simulink model "controller"  (R2024b)
settings: Solver=FixedStepDiscrete  StartTime=0.0  StopTime=10  FixedStep=1/10  RelTol=1e-3
undefined symbols (not defined in the file or in its folder): MAX_TORQUE, MAX_TORQUE_REVERSE
settings Model: ExtModeTrigDuration=2  Creator=DAUIN-Win10  LastModifiedBy=yoyom
settings SolverCC: AutoInsertRateTranBlk=on
settings OptimizationCC: EnhancedBackFolding=on  PassReuseOutputArgsAs=Individual arguments  ZeroExternalMemoryAtStartup=off  ZeroInternalMemoryAtStartup=off  MaxStackSize=64  OptimizeBlockOrder=speed  DifferentSizesBufferReuse=on  OptimizationCustomize=off  EfficientTunableParamExpr=on
settings DebuggingCC: ParameterTunabilityLossMsg=error  UnconnectedInputMsg=warning  UnconnectedOutputMsg=warning  UnconnectedLineMsg=warning
settings HardwareCC: ProdBitPerInt=16  ProdBitPerPointer=16  ProdBitPerSizeT=16  ProdBitPerPtrDiffT=16  ProdLargestAtomicFloat=None  ProdWordSize=8  ProdHWDeviceType=Atmel->AVR
settings ModelReferenceCC: EnableRefExpFcnMdlSchedulingChecks=on
settings SFSimCC: MATLABDynamicMemAlloc=off
settings RTWCC: Description=Embedded Coder  SystemTargetFile=ert.tlc  HardwareBoard=Arduino Uno  TemplateMakefile=ert_default_tmf  Toolchain=Arduino AVR  BuildConfiguration=Faster Runs  GPUComputeCapability=3.5  DLArmComputeVersion=19.05
settings CodeAppCC: ForceParamTrailComments=on  IgnoreCustomStorageClasses=off  OperatorAnnotations=on  SimulinkDataObjDesc=on  SFDataObjDesc=on  InsertBlockDesc=on
settings ERTTargetCC: SupportContinuousTime=on  SupportNonInlinedSFcns=on  SupportVariableSizeSignals=on  ExtModeTransport=3  ExtModeStaticAlloc=on  ExtModeAutomaticAllocSize=off  ExtModeStaticAllocSize=250  ExtModeMexFile=ext_xcp  ExtModeIntrfLevel=Level2 - Open  InlinedParameterPlacement=Hierarchical  ERTFilePackagingFormat=Compact

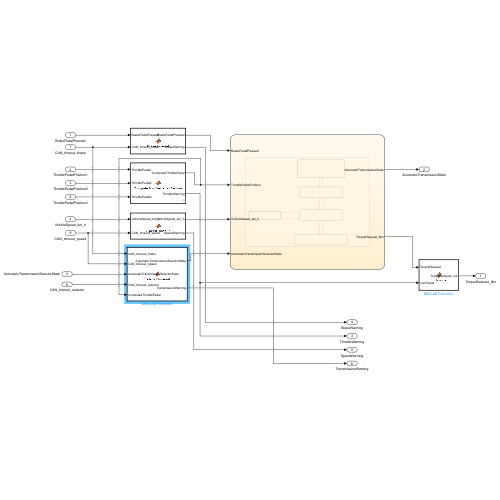
[thumbnail: Simulink's stored preview of the top-level diagram]
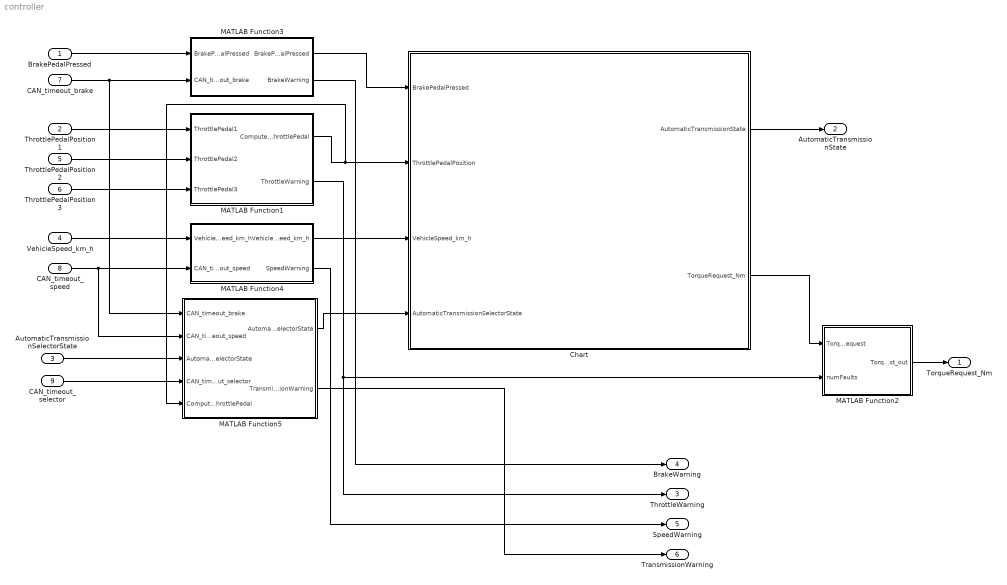
== system controller ==
  BrakePedalPressed : Inport  OutDataTypeStr=boolean
  ThrottlePedalPosition1 : Inport  Port=2  OutDataTypeStr=single
  AutomaticTransmissionSelectorState : Inport  Port=3  OutDataTypeStr=Enum: TransmissionState
  VehicleSpeed_km_h : Inport  Port=4  OutDataTypeStr=single  Unit=km/h
  ThrottlePedalPosition2 : Inport  Port=5  OutDataTypeStr=single
  ThrottlePedalPosition3 : Inport  Port=6  OutDataTypeStr=single
  CAN_timeout_brake : Inport  Port=7
  CAN_timeout_speed : Inport  Port=8
  CAN_timeout_selector : Inport  Port=9
  Chart : Stateflow chart  TreatAsAtomicUnit=on
  MATLAB Function1 : MATLAB Function  TreatAsAtomicUnit=on
  MATLAB Function2 : MATLAB Function  TreatAsAtomicUnit=on
  MATLAB Function3 : MATLAB Function  TreatAsAtomicUnit=on
  MATLAB Function4 : MATLAB Function  TreatAsAtomicUnit=on
  MATLAB Function5 : MATLAB Function  TreatAsAtomicUnit=on
  TorqueRequest_Nm : Outport  OutDataTypeStr=single  Unit=N*m
  AutomaticTransmissionState : Outport  Port=2  OutDataTypeStr=Enum: TransmissionState
  ThrottleWarning : Outport  Port=3  OutDataTypeStr=single  Unit=N*m
  BrakeWarning : Outport  Port=4  OutDataTypeStr=single  Unit=N*m
  SpeedWarning : Outport  Port=5  OutDataTypeStr=single  Unit=N*m
  TransmissionWarning : Outport  Port=6  OutDataTypeStr=single  Unit=N*m
  wires:
  Chart/2(TorqueRequest_Nm) -> MATLAB Function2/1(TorqueRequest)
  Chart/1(AutomaticTransmissionState) -> AutomaticTransmissionState/1
  BrakePedalPressed/1 -> MATLAB Function3/1("BrakePedalPressed ")
  AutomaticTransmissionSelectorState/1 -> MATLAB Function5/3("AutomaticTransmissionSelectorState ")
  VehicleSpeed_km_h/1 -> MATLAB Function4/1("VehicleSpeed_km_h ")
  MATLAB Function1/2(ThrottleWarning) -> MATLAB Function2/2(numFaults), ThrottleWarning/1
  MATLAB Function2/1(TorqueRequest_out) -> TorqueRequest_Nm/1
  ThrottlePedalPosition1/1 -> MATLAB Function1/1(ThrottlePedal1)
  ThrottlePedalPosition3/1 -> MATLAB Function1/3(ThrottlePedal3)
  ThrottlePedalPosition2/1 -> MATLAB Function1/2(ThrottlePedal2)
  CAN_timeout_brake/1 -> MATLAB Function5/1(CAN_timeout_brake), MATLAB Function3/2(CAN_timeout_brake)
  CAN_timeout_speed/1 -> MATLAB Function5/2(CAN_timeout_speed), MATLAB Function4/2(CAN_timeout_speed)
  MATLAB Function3/1(BrakePedalPressed) -> Chart/1(BrakePedalPressed)
  MATLAB Function1/1(ComputedThrottlePedal) -> MATLAB Function5/5(ComputedThrottlePedal), Chart/2(ThrottlePedalPosition)
  MATLAB Function4/1(VehicleSpeed_km_h) -> Chart/3(VehicleSpeed_km_h)
  MATLAB Function5/2(TransmissionWarning) -> TransmissionWarning/1
  MATLAB Function4/2(SpeedWarning) -> SpeedWarning/1
  MATLAB Function3/2(BrakeWarning) -> BrakeWarning/1
  MATLAB Function5/1(AutomaticTransmissionSelectorState) -> Chart/4(AutomaticTransmissionSelectorState)
  CAN_timeout_selector/1 -> MATLAB Function5/4(CAN_timeout_selector)

== matlab function controller/MATLAB Function2 ==
  data: TorqueRequest input; numFaults input; TorqueRequest_out output
function TorqueRequest_out = fcnTorque(TorqueRequest, numFaults)
    if(numFaults==2)
        TorqueRequest_out = single(0);
    else
        TorqueRequest_out = TorqueRequest;
    end

== stateflow chart controller/Chart ==
  state Situations [parallel]
    settings: executionOrder=1
    state Brake
      entry:
      AutomaticTransmissionState = TransmissionState.Brake;
      during:
      if (ThrottlePedalPosition >= 0 && ThrottlePedalPosition <= (1/3))
      if (VehicleSpeed_km_h<=0)
      TorqueRequest_Nm=0;
      else
      TorqueRequest_Nm = -(-3 * ThrottlePedalPosition + 1) * MAX_TORQUE;
      end
      else
      TorqueRequest_Nm = ((3/2) * ThrottlePedalPosition - (1/2)) * MAX_TORQUE;
      end
    state Drive
      entry:
      AutomaticTransmissionState = TransmissionState.Drive;
      during:
      TorqueRequest_Nm = ThrottlePedalPosition*MAX_TORQUE;
    state Neutral
      entry:
      TorqueRequest_Nm = 0;
      AutomaticTransmissionState = TransmissionState.Neutral;
    state Park
      entry:
      TorqueRequest_Nm = 0;
      AutomaticTransmissionState = TransmissionState.Park;
    state Reverse
      entry:
      AutomaticTransmissionState = TransmissionState.Reverse;
      during:
      TorqueRequest_Nm = -ThrottlePedalPosition*MAX_TORQUE_REVERSE;
    Brake -> Drive : [ AutomaticTransmissionSelectorState == TransmissionState.Drive || ...
        | AutomaticTransmissionSelectorState == TransmissionState.Neutral || ...
        | AutomaticTransmissionSelectorState == TransmissionState.Reverse || ...
        | AutomaticTransmissionSelectorState == TransmissionState.Park ]
    Drive -> Brake [order 2] : [ThrottlePedalPosition>1/3 && ...
        | AutomaticTransmissionSelectorState == TransmissionState.Brake]
    Drive -> Neutral [order 1] : [ AutomaticTransmissionSelectorState == TransmissionState.Neutral || ...
        | AutomaticTransmissionSelectorState == TransmissionState.Park || ...
        | AutomaticTransmissionSelectorState == TransmissionState.Reverse ]
    Neutral -> Drive [order 1] : [ VehicleSpeed_km_h > -5 && BrakePedalPressed == true && ...
        | ( AutomaticTransmissionSelectorState == TransmissionState.Drive || ...
        | AutomaticTransmissionSelectorState == TransmissionState.Brake ) ]
    (default) -> Park
    Neutral -> Park [order 3] : [ abs(VehicleSpeed_km_h) < 5 && BrakePedalPressed == true && ...
        | AutomaticTransmissionSelectorState == TransmissionState.Park ]
    Park -> Neutral : [BrakePedalPressed == true && ...
        | (AutomaticTransmissionSelectorState == TransmissionState.Neutral || ...
        | AutomaticTransmissionSelectorState == TransmissionState.Drive || ...
        | AutomaticTransmissionSelectorState == TransmissionState.Brake || ...
        | AutomaticTransmissionSelectorState == TransmissionState.Reverse)]
    Neutral -> Reverse [order 2] : [ VehicleSpeed_km_h < 5 && BrakePedalPressed==true && ...
        | AutomaticTransmissionSelectorState == TransmissionState.Reverse ]
    Reverse -> Neutral : [ AutomaticTransmissionSelectorState == TransmissionState.Neutral || ...
        | AutomaticTransmissionSelectorState == TransmissionState.Drive || ...
        | AutomaticTransmissionSelectorState == TransmissionState.Brake || ...
        | AutomaticTransmissionSelectorState == TransmissionState.Park ]
  data: BrakePedalPressed input boolean; ThrottlePedalPosition input single; VehicleSpeed_km_h input single; AutomaticTransmissionState output Enum: TransmissionState; TorqueRequest_Nm output single; MAX_TORQUE parameter single; MAX_TORQUE_REVERSE parameter single; AutomaticTransmissionSelectorState input Enum: TransmissionState

== matlab function controller/MATLAB Function3 ==
  data: BrakePedalPressed input; CAN_timeout_brake input boolean; BrakePedalPressed output; BrakeWarning output single
function [BrakePedalPressed, BrakeWarning] = BrakeTimeout(BrakePedalPressed, CAN_timeout_brake)    
    if(CAN_timeout_brake==true)
        BrakePedalPressed=true;
        BrakeWarning=single(3);
    else
        BrakeWarning=single(0);
    end

== matlab function controller/MATLAB Function4 ==
  data: VehicleSpeed_km_h input; CAN_timeout_speed input boolean; VehicleSpeed_km_h output; SpeedWarning output single
function [VehicleSpeed_km_h, SpeedWarning]= SpeedTimeout(VehicleSpeed_km_h, CAN_timeout_speed)    
    if(CAN_timeout_speed==true)
        VehicleSpeed_km_h=single(0);
        SpeedWarning=single(4);
    else
        SpeedWarning=single(0);
    end

== matlab function controller/MATLAB Function5 ==
  data: CAN_timeout_brake input; CAN_timeout_speed input; AutomaticTransmissionSelectorState output; AutomaticTransmissionSelectorState input; CAN_timeout_selector input boolean; TransmissionWarning output single; ComputedThrottlePedal input
function [AutomaticTransmissionSelectorState, TransmissionWarning] = SelectorTimeout(CAN_timeout_brake, CAN_timeout_speed, AutomaticTransmissionSelectorState, CAN_timeout_selector, ComputedThrottlePedal)    
    if(CAN_timeout_selector==true)
        TransmissionWarning = single(5);
        AutomaticTransmissionSelectorState = TransmissionState.Drive;
        if(CAN_timeout_speed==true || CAN_timeout_brake==true)
            AutomaticTransmissionSelectorState = TransmissionState.Drive;
        end
    else
        TransmissionWarning = single(0);
        end
    if(ComputedThrottlePedal==single(-1))
        AutomaticTransmissionSelectorState = TransmissionState.Neutral;
    end

== matlab function controller/MATLAB Function1 ==
  data: ThrottlePedal1 input; ThrottlePedal2 input; ThrottlePedal3 input; ComputedThrottlePedal output single; ThrottleWarning output single
function [ComputedThrottlePedal,ThrottleWarning] = ComputeThrottlePedalPosition(ThrottlePedal1, ThrottlePedal2, ThrottlePedal3)
    tol = 0.05;
    ThrottleWarning=single(0);
    
    if(abs(ThrottlePedal1-ThrottlePedal2)<tol)
        if(abs(ThrottlePedal1-ThrottlePedal3)<tol && abs(ThrottlePedal2-ThrottlePedal3)<tol)
            ComputedThrottlePedal = mean([ThrottlePedal1 ThrottlePedal2 ThrottlePedal3]);
        else 
            ComputedThrottlePedal = mean([ThrottlePedal1 ThrottlePedal2]);
            ThrottleWarning = single(1);
        end
    elseif(abs(ThrottlePedal1-ThrottlePedal3)<tol)
            ComputedThrottlePedal = mean([ThrottlePedal1 ThrottlePedal3]);
            ThrottleWarning = single(1);
    elseif(abs(ThrottlePedal2-ThrottlePedal3)<tol)
            ComputedThrottlePedal = mean([ThrottlePedal2 ThrottlePedal3]);
            ThrottleWarning = single(1);
    else
        ThrottleWarning = single(2);
        ComputedThrottlePedal = single(-1);
    end
